simulink model "radar_switch"  (Simulink 8.2)
settings: Solver=ode1  StartTime=0.0  StopTime=Inf  FixedStep=0.001  RelTol=1e-3
PostLoadFcn:
  | , if any(exist('dsrtsu_mdlpostloadfcn', 'file') == [2, 3, 6]), try dsrtsu_mdlpostloadfcn('Execute', bdroot); catch fprintf('Error in PostLoadFcn (dsrtsu_mdlpostloadfcn) for model "%s":\n %s\n', bdroot, lasterr); end, end,
libraries: simulink x2
settings Model: DSRTSU_INTERNAL_RTI_VER=450  DSRTSU_INTERNAL_RTI_TYPE=rti1401  Creator=rushk1  LastModifiedBy=rushk1  BufferReuse=off
settings DataIOCC: SignalLoggingSaveFormat=Dataset
settings OptimizationCC: BlockReduction=off  OptimizeBlockIOStorage=off  BufferReuse=off  ExpressionFolding=off  ExpressionDepthLimit=128  LocalBlockOutputs=off
settings DebuggingCC: FcnCallInpInsideContextMsg=EnableAllAsError  StateNameClashWarn=none
settings RTWCC: SystemTargetFile=rti1401.tlc  MakeCommand=make_rti  TemplateMakefile=rti1401.tmf  Description=dSPACE DS1401 Hardware Platform  ProcessScript=rti1401_make_rtw_hook
settings STFCustomTargetCC: CodeReplacementLibrary=ANSI_C  ModelReferenceCompliant=off  ParMdlRefBuildCompliant=on  GeneratePreprocessorConditionals=Disable all  MatFileLogging=on  SystemTargetFile=rti1401.tlc
settings GRTTargetCC: ModelReferenceCompliant=off  CompOptLevelCompliant=off  ConcurrentExecutionCompliant=off
settings CustomProperty: DataType=RTWOptions_EnumType_C__Program Files_dSPACE RCPHIL 2014-B_MATLAB_RTI_RTI1401_TLC_rti1401_1InitialSimState  Value=RUN
settings EnumStrPairs: String=RUN

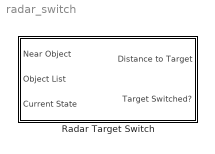
== system radar_switch ==
  Radar Target Switch : Subsystem

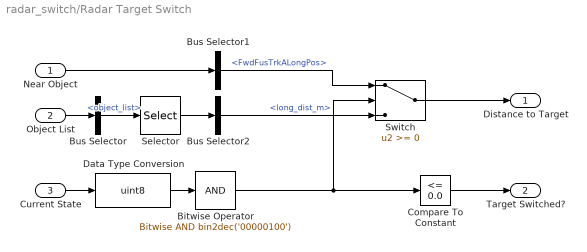
== system radar_switch/Radar Target Switch ==
  Near Object : Inport  OutDataTypeStr=Bus: FusObjectTrackA
  Object List : Inport  Port=2  OutDataTypeStr=Bus: FusObjectList
  Current State : Inport  Port=3
  Bitwise Operator : simulink/Logic and Bit Operations/Bitwise Operator  logicop=AND  UseBitMask=on  BitMask=bin2dec('00000100')  BitMaskRealWorld=Stored Integer
  Bus Selector : BusSelector  OutputSignals=object_list
  Bus Selector1 : BusSelector  OutputSignals=FwdFusTrkALongPos
  Bus Selector2 : BusSelector  OutputSignals=long_dist_m
  Compare To Constant : simulink/Logic and Bit Operations/Compare To Constant  relop=<=  const=0.0  OutDataTypeStr=boolean
  Data Type Conversion : DataTypeConversion  OutDataTypeStr=uint8
  Selector : Selector  InputPortWidth=4  IndexOptions=Index vector (dialog)  Indices=[2]  OutputSizes=1
  Switch : Switch
  Distance to Target : Outport
  Target Switched? : Outport  Port=2
  wires:
  Switch/1 -> Distance to Target/1
  Object List/1 -> Bus Selector/1
  Bus Selector/1 -> Selector/1  "<object_list>"
  Bitwise Operator/1 -> Compare To Constant/1, Switch/2
  Current State/1 -> Data Type Conversion/1
  Near Object/1 -> Bus Selector1/1
  Bus Selector1/1 -> Switch/1  "<FwdFusTrkALongPos>"
  Selector/1 -> Bus Selector2/1
  Bus Selector2/1 -> Switch/3  "<long_dist_m>"
  Data Type Conversion/1 -> Bitwise Operator/1
  Compare To Constant/1 -> Target Switched?/1
